simulink model "encoder_hall_block2"  (R2012b)
settings: Solver=ode45  StartTime=0.0  StopTime=1  RelTol=1e-3
libraries: BLDC x1, Encoder x1
settings Model: Creator=h3now  LastModifiedBy=h3now

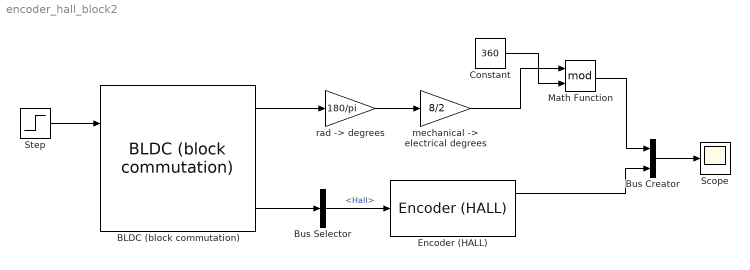
== system encoder_hall_block2 ==
  BLDC (block commutation) : BLDC/BLDC (block commutation)  J=1.39e-6  R=10.1/2  L=2.04/2000  P=8  Kt=15.7e-3/1.19  Ke=15.7e-3/1.19  Kd=0
  Bus Creator : BusCreator  Inputs=2
  Bus Selector : BusSelector  OutputSignals=Hall
  Constant : Constant  Value=360
  Encoder (HALL) : Encoder/Encoder (HALL)
  Math Function : Math  Operator=mod  SaturateOnIntegerOverflow=on
  Scope : Scope
  Step : Step  Time=0.3  Before=4  After=0  SampleTime=0
  "mechanical -> electrical degrees" : Gain  Gain=8/2
  "rad -> degrees" : Gain  Gain=180/pi
  wires:
  Step/1 -> BLDC (block commutation)/1
  BLDC (block commutation)/3 -> Bus Selector/1
  Bus Selector/1 -> Encoder (HALL)/1  "<Hall>"
  Bus Creator/1 -> Scope/1
  BLDC (block commutation)/1 -> "rad -> degrees"/1
  "rad -> degrees"/1 -> "mechanical -> electrical degrees"/1
  "mechanical -> electrical degrees"/1 -> Math Function/1
  Constant/1 -> Math Function/2
  Math Function/1 -> Bus Creator/1
  Encoder (HALL)/1 -> Bus Creator/2
